simulink model "Vehicle_Model_WIP_V2"  (R2019b)
settings: Solver=FixedStepDiscrete  StartTime=0.0  StopTime=Simulink.t_end  FixedStep=Simulink.dt  RelTol=1e-3
undefined symbols (not defined in the file): BRK, BTRRAD, CHLR, CHRG, DCDC, DiscIntNeverNeededParam, FAN, INV, MTR, PTRAD, PUMP, Settings, TRSM, Vehicle, VHCL, WHL
libraries: simulink x9, EV_cooling x6, EV_VLD x5, EV_ePWT x5
(part 5 of 5)

== system Vehicle_Model_WIP_V2/old cooling/Fan and air for Radiators/Air Flow and Fan Model/Fan Inertia ==
  Max Volumetric flow rate [lpm : Inport
  Discrete-Time Integrator : DiscreteIntegrator  SampleTime=-1  ICPrevOutput=DiscIntNeverNeededParam  ICPrevScaledInput=DiscIntNeverNeededParam
  Divide6 : Product  Inputs=*/
  Divide7 : Product  Inputs=*/
  Divide8 : Product  Inputs=/*
  Subtract : Sum  Inputs=+-
  Tau : Constant  Value=3
  one : Constant
  RAD_dVFan_m3ph : Outport
  wires:
  Discrete-Time Integrator/1 -> RAD_dVFan_m3ph/1, Divide7/1
  Divide8/1 -> Divide6/2
  Tau/1 -> Divide7/2, Divide8/2
  Max Volumetric flow rate [lpm/1 -> Divide6/1
  one/1 -> Divide8/1
  Divide6/1 -> Subtract/1
  Subtract/1 -> Discrete-Time Integrator/1
  Divide7/1 -> Subtract/2

== system Vehicle_Model_WIP_V2/old cooling/Fan and air for Radiators/Air Flow and Fan Model/If Action Subsystem ==
  In1 : Inport
  Action Port : ActionPort  ActionPortLabel=if(u1 == 1)
  Out1 : Outport
  wires:
  In1/1 -> Out1/1

== system Vehicle_Model_WIP_V2/old cooling/Fan and air for Radiators/Air Flow and Fan Model/If Action Subsystem1 ==
  In1 : Inport
  Action Port : ActionPort  ActionPortLabel=else
  Out1 : Outport
  wires:
  In1/1 -> Out1/1

== system Vehicle_Model_WIP_V2/old cooling/PowerTrain Cooling system/Low Temperature Radiator/Radiator Thermal model  ==
  RADBCS_TAirOut_degC : Inport
  RAD_TWtrIn_degC : Inport  Port=2
  RAD_dmAir_kgps : Inport  Port=3
  RAD_dmWtr_kgps : Inport  Port=4
  RAD_UA_WpK : Inport  Port=5
  Air Heat Capacity J/kgK : Lookup_n-D  NumberOfTableDimensions=1  BreakpointsForDimension1=[-40 -30 -20 -10 0 5 10 15 20 25 30 35 40 45 50 60 70 80 90 100]  Table=[1002 1004 1005 1006 1006 1007 1008 1009 1010 1011 1011 1012 1013 1014 1016 1017 1019 1020 1021 1022]  ExtrapMethod=Clip  RndMeth=Simplest  InputSameDT=on
  Constant : Constant  Value=-1
  Constant{1..3,7} (4 alike) : Constant
  Constant4 : Constant  Value=-1
  Constant6 : Constant  Value=-1
  Delay : Delay  DelayLength=1  InitialConditionSource=Input port
      settings: InputPortMap=u0,p4
  Delay1 : Delay  InitialConditionSource=Input port
      settings: InputPortMap=u0,p4
  Divide{1,3,8,10,12,15} (6 alike) : Product  Inputs=*/
  Divide{2,4..7,9,11,13..14,16} (10 alike) : Product  Inputs=**
  Exp : Math  SignedPower=off  SaturateOnIntegerOverflow=on
  Exp1 : Math  SignedPower=off  SaturateOnIntegerOverflow=on
  Exp2 : Math  SignedPower=off  SaturateOnIntegerOverflow=on
  Gain : Gain  Gain=0.5
  Heat Capacity  Water-Glycol 80-20%vol J/kgK : Lookup_n-D  NumberOfTableDimensions=1  BreakpointsForDimension1=[-45.56 -17.78 10 37.77 65.55 93.33 121.11 148.88 176.66]  Table="[3841.6 3888.1  3934.6 3981.1 4027.6 4074.0 4120.5 4167.0 4213.6]"  ExtrapMethod=Clip  RndMeth=Simplest  InputSameDT=on
  If Action Subsystem1 : Subsystem  Commented=on  TreatAsAtomicUnit=on
  Subtract{1..7} (7 alike) : Sum  Inputs=+-
  Subtract8 : Sum
  RAD_TAirOut_degC : Outport  VectorParamsAs1DForOutWhenUnconnected=off
  RAD_TWtrOut_degC : Outport  Port=2  VectorParamsAs1DForOutWhenUnconnected=off
  RAD_TWtrBlk_degC : Outport  Port=3  VectorParamsAs1DForOutWhenUnconnected=off
  RAD_PHeatRej_W : Outport  Port=4  VectorParamsAs1DForOutWhenUnconnected=off
  wires:
  [RAD_TWtrBlk_degC] -> RAD_TWtrBlk_degC/1
  [RAD_TAirOut_degC] -> RAD_TAirOut_degC/1
  [RAD_TWtrOut_degC] -> RAD_TWtrOut_degC/1
  Heat Capacity  Water-Glycol 80-20%vol J/kgK/1 -> [RAD_cpWtr]
  [RAD_TWtrBlk_degC] -> Heat Capacity  Water-Glycol 80-20%vol J/kgK/1
  [RAD_TAirBlk_degC] -> Air Heat Capacity J/kgK/1
  Air Heat Capacity J/kgK/1 -> [RAD_cpAir]
  [RAD_PHeatRej_W] -> RAD_PHeatRej_W/1
  RAD_UA_WpK/1 -> [RAD_UA_WpK]
  RAD_dmAir_kgps/1 -> [RAD_dmAir_kgps]
  RAD_dmWtr_kgps/1 -> [RAD_dmWtr_kgps]
  RADBCS_TAirOut_degC/1 -> [RADBCS_TAirOut_degC]
  RAD_TWtrIn_degC/1 -> [RAD_TWtrIn_degC]
  [RAD_PHeatRej_W] -> Divide13/2
  [RAD_dmWtr_kgps] -> Divide6/1
  Divide9/1 -> [RAD_PHeatRej_W]
  Exp/1 -> Subtract2/2
  [RAD_TAirBlk_degC] -> Subtract5/1
  Divide13/1 -> Subtract5/2
  [tauWtr] -> Divide8/2
  Subtract3/1 -> Divide11/1
  [RAD_TAirBlk_degC] -> Subtract1/1
  Exp1/1 -> Divide11/2
  Constant7/1 -> Divide12/1
  [RAD_TAirBlk_degC] -> Subtract3/1
  Constant2/1 -> Subtract2/1
  Subtract1/1 -> Divide7/2
  [RAD_TWtrIn_degC] -> Subtract1/2
  Constant6/1 -> Divide10/1
  Divide5/1 -> [tauWtr]
  [RAD_TAirBlk_degC] -> Subtract4/1
  [RAD_UA_WpK] -> Divide12/2
  Subtract4/1 -> [RAD_TWtrOut_degC]
  [tauWtr] -> Divide10/2
  Divide3/1 -> Divide5/2
  Divide11/1 -> Subtract4/2
  Divide10/1 -> Exp1/1
  Divide2/1 -> Divide5/1
  [RAD_TWtrIn_degC] -> Delay/2
  Subtract2/1 -> Divide9/2
  Constant/1 -> Divide8/1
  Divide6/1 -> Divide7/1
  Divide7/1 -> Divide9/1
  Divide8/1 -> Exp/1
  [RAD_dmWtr_kgps] -> Divide2/1
  [RAD_cpWtr] -> Divide2/2
  Subtract5/1 -> Delay/1
  [RAD_cpWtr] -> Divide6/2
  [RAD_TWtrIn_degC] -> Subtract3/2
  Divide12/1 -> Divide13/1
  Delay/1 -> [RAD_TWtrBlk_degC]
  [RAD_UA_WpK] -> Divide3/2
  Constant3/1 -> Divide3/1
  Constant1/1 -> Divide15/1
  [RAD_UA_WpK] -> Divide15/2
  [RADBCS_TAirOut_degC] -> Subtract6/2
  [RAD_cpAir] -> Divide14/2
  [RAD_dmAir_kgps] -> Divide14/1
  Divide14/1 -> Divide16/1
  Divide1/1 -> Exp2/1
  Divide4/1 -> Subtract7/2
  Divide15/1 -> Divide16/2
  [tauAir] -> Divide1/2
  Subtract7/1 -> [RAD_TAirOut_degC]
  [RAD_TWtrBlk_degC] -> Subtract7/1
  Divide16/1 -> [tauAir]
  Constant4/1 -> Divide1/1
  [RAD_TWtrBlk_degC] -> Subtract6/1
  Exp2/1 -> Divide4/2
  Subtract6/1 -> Divide4/1
  Delay1/1 -> [RAD_TAirBlk_degC]
  [RADBCS_TAirOut_degC] -> Subtract8/1
  [RAD_TAirOut_degC] -> Subtract8/2
  Subtract8/1 -> Gain/1
  [RADBCS_TAirOut_degC] -> Delay1/2
  Gain/1 -> Delay1/1

== system Vehicle_Model_WIP_V2/VLD/old/OLD VLD/Vehicle Longitudinal Dinamic  Model (No Slip)/Wheel speed Front ==
  Vehicle Actual Speed [km/h] : Inport
  VLD_RWhlFr_m : Inport  Port=2
  Constant : Constant  Value=3.6
  Constant1 : Constant  Value=60
  Constant2 : Constant  Value=pi()
  Constant3 : Constant  Value=2
  Constant4 : Constant
  Divide : Product  Inputs=*/
  Divide1 : Product  Inputs=*/
  Divide2 : Product
  Divide3 : Product  Inputs=*/
  Divide4 : Product
  Max : MinMax  Function=max  Inputs=2
  VLD_nWhlFr_rpm : Outport  VectorParamsAs1DForOutWhenUnconnected=off
  VLD_vWhlFr_mps : Outport  Port=2
  wires:
  Divide/1 -> Divide1/1, [VLD_vWhlFr_mps]
  [VLD_vWhlFr_mps] -> VLD_vWhlFr_mps/1
  VLD_RWhlFr_m/1 -> [VLD_RWhlFr_m]
  Vehicle Actual Speed [km/h]/1 -> [Vehicle_Actual_Speed_kph]
  [Vehicle_Actual_Speed_kph] -> Divide/1
  Constant/1 -> Divide/2
  [VLD_RWhlFr_m] -> Divide1/2
  Divide1/1 -> Divide2/1
  Constant1/1 -> Divide2/2
  Divide2/1 -> Divide3/1
  Divide4/1 -> Divide3/2
  Constant3/1 -> Divide4/1
  Constant2/1 -> Divide4/2
  Divide3/1 -> Max/1
  [VLD_nWhlFr_rpm] -> VLD_nWhlFr_rpm/1
  Max/1 -> [VLD_nWhlFr_rpm]
  Constant4/1 -> Max/2

== system Vehicle_Model_WIP_V2/VLD/old/OLD VLD/Vehicle Longitudinal Dinamic  Model (No Slip)/Wheel speed Rear ==
  Vehicle Actual Speed [km/h] : Inport
  VLD_RWhlRr_m : Inport  Port=2
  Constant : Constant  Value=3.6
  Constant1 : Constant  Value=60
  Constant2 : Constant  Value=pi()
  Constant3 : Constant  Value=2
  Constant4 : Constant
  Divide : Product  Inputs=*/
  Divide1 : Product  Inputs=*/
  Divide2 : Product
  Divide3 : Product  Inputs=*/
  Divide4 : Product
  Max : MinMax  Function=max  Inputs=2
  LVD_nWhlRr_rpm : Outport  VectorParamsAs1DForOutWhenUnconnected=off
  VLD_vWhlRr_mps : Outport  Port=2
  wires:
  [VLD_vWhlRr_mps] -> VLD_vWhlRr_mps/1
  Constant4/1 -> Max/2
  [VLD_nWhlRr_rpm] -> LVD_nWhlRr_rpm/1
  Divide3/1 -> Max/1
  Constant2/1 -> Divide4/2
  Constant3/1 -> Divide4/1
  Divide4/1 -> Divide3/2
  Divide2/1 -> Divide3/1
  Constant1/1 -> Divide2/2
  Divide1/1 -> Divide2/1
  [VLD_RWhlRr_m] -> Divide1/2
  Divide/1 -> Divide1/1, [VLD_vWhlRr_mps]
  Constant/1 -> Divide/2
  [Vehicle_Actual_Speed_kph] -> Divide/1
  Vehicle Actual Speed [km/h]/1 -> [Vehicle_Actual_Speed_kph]
  VLD_RWhlRr_m/1 -> [VLD_RWhlRr_m]
  Max/1 -> [VLD_nWhlRr_rpm]

== system Vehicle_Model_WIP_V2/VLD/old/OLD VLD/Vehicle Longitudinal Dinamic Model (Slip)/Slip Model Front ==
  VLD_vWhl_mps : Inport
  VLD_vVhcl_mps : Inport  Port=2
  Abs : Abs
  Constant3 : Constant  Value=1e-3
  Gain : Gain  Gain=3.6
  Gain1 : Gain  Gain=3.6
  If : If  IfExpression=u1 == 1
  If Action Subsystem : Subsystem  TreatAsAtomicUnit=on
  If Action Subsystem1 : Subsystem  TreatAsAtomicUnit=on
  Merge : Merge
  Relational Operator2 : RelationalOperator  Operator=>  OutDataTypeStr=boolean  RndMeth=Simplest
  Saturatio1 : Saturate  UpperLimit=inf  LowerLimit=1e-3
  Saturatio2 : Saturate  UpperLimit=inf  LowerLimit=1e-3
  Saturatio3 : Saturate  UpperLimit=1  LowerLimit=-1
  Scope2 : Scope
  Slip Calculation2 : Subsystem  Commented=on
  Slip Calculation3 : Subsystem
  Zero : Constant  Value=0  OutDataTypeStr=Inherit: Inherit via back propagation
  slip : Outport
  wires:
  [VLD_rSlip] -> slip/1
  [VLD_vVhcl_mps] -> Gain1/1
  If/2 -> If Action Subsystem1/Action
  Saturatio1/1 -> Slip Calculation3/1(w)
  Saturatio2/1 -> Slip Calculation3/2(v)
  If Action Subsystem/1(Out1) -> Merge/1
  Merge/1 -> Saturatio3/1
  Constant3/1 -> Relational Operator2/2
  Relational Operator2/1 -> If/1
  If Action Subsystem1/1(Out1) -> Merge/2
  Abs/1 -> Relational Operator2/1
  Zero/1 -> If Action Subsystem1/1(In1)  "slip"
  [VLD_vWhl_mps] -> Abs/1, Gain/1
  If/1 -> If Action Subsystem/Action
  Slip Calculation3/1(slip) -> If Action Subsystem/1(In1)
  VLD_vVhcl_mps/1 -> [VLD_vVhcl_mps]
  VLD_vWhl_mps/1 -> [VLD_vWhl_mps]
  Saturatio3/1 -> [VLD_rSlip], Scope2/1
  Gain/1 -> Saturatio1/1
  Gain1/1 -> Saturatio2/1

== system Vehicle_Model_WIP_V2/VLD/old/OLD VLD/Vehicle Longitudinal Dinamic Model (Slip)/Slip Model Rear ==
  VLD_vWhl_mps : Inport
  VLD_vVhcl_mps : Inport  Port=2
  Abs : Abs
  Constant3 : Constant  Value=1e-3
  Gain1 : Gain  Gain=3.6
  Gain2 : Gain  Gain=3.6
  If : If  IfExpression=u1 == 1
  If Action Subsystem : Subsystem  TreatAsAtomicUnit=on
  If Action Subsystem1 : Subsystem  TreatAsAtomicUnit=on
  Merge : Merge
  Relational Operator2 : RelationalOperator  Operator=>  OutDataTypeStr=boolean  RndMeth=Simplest
  Saturatio1 : Saturate  UpperLimit=inf  LowerLimit=1e-3
  Saturatio2 : Saturate  UpperLimit=inf  LowerLimit=1e-3
  Scope2 : Scope
  Scope3 : Scope
  Scope6 : Scope
  Slip Calculation2 : Subsystem  Commented=on
  Slip Calculation3 : Subsystem
  Zero : Constant  Value=0  OutDataTypeStr=Inherit: Inherit via back propagation
  slip : Outport
  wires:
  VLD_vWhl_mps/1 -> [VLD_vWhl_mps]
  VLD_vVhcl_mps/1 -> [VLD_vVhcl_mps]
  Slip Calculation3/1(slip) -> If Action Subsystem/1(In1), Scope3/1
  If/1 -> If Action Subsystem/Action
  [VLD_vWhl_mps] -> Abs/1, Gain1/1
  Zero/1 -> If Action Subsystem1/1(In1)  "slip"
  Abs/1 -> Relational Operator2/1
  If Action Subsystem1/1(Out1) -> Merge/2
  Relational Operator2/1 -> If/1, Scope6/1
  Constant3/1 -> Relational Operator2/2
  If Action Subsystem/1(Out1) -> Merge/1
  Saturatio2/1 -> Slip Calculation3/2(v)
  Saturatio1/1 -> Slip Calculation3/1(w)
  If/2 -> If Action Subsystem1/Action
  [VLD_vVhcl_mps] -> Gain2/1
  [VLD_rSlip] -> slip/1
  Merge/1 -> [VLD_rSlip], Scope2/1
  Gain1/1 -> Saturatio1/1
  Gain2/1 -> Saturatio2/1

== system Vehicle_Model_WIP_V2/VLD/old/OLD VLD/Vehicle Longitudinal Dinamic Model (Slip)/Subsystem2 ==
  rad/s : Inport
  Constant1 : Constant  Value=60
  Constant2 : Constant  Value=pi()
  Constant3 : Constant  Value=2
  Divide2 : Product
  Divide3 : Product  Inputs=*/
  Divide4 : Product
  rpm : Outport
  wires:
  rad/s/1 -> Divide2/1
  Constant2/1 -> Divide4/2
  Divide2/1 -> Divide3/1
  Divide3/1 -> rpm/1
  Constant1/1 -> Divide2/2
  Divide4/1 -> Divide3/2
  Constant3/1 -> Divide4/1

== system Vehicle_Model_WIP_V2/VLD/old/OLD VLD/Vehicle Longitudinal Dinamic Model (Slip)/Subsystem3 ==
  rad/s : Inport
  Constant1 : Constant  Value=60
  Constant2 : Constant  Value=pi()
  Constant3 : Constant  Value=2
  Divide2 : Product
  Divide3 : Product  Inputs=*/
  Divide4 : Product
  rpm : Outport
  wires:
  Constant3/1 -> Divide4/1
  Divide4/1 -> Divide3/2
  Constant1/1 -> Divide2/2
  Divide3/1 -> rpm/1
  Divide2/1 -> Divide3/1
  Constant2/1 -> Divide4/2
  rad/s/1 -> Divide2/1

== system Vehicle_Model_WIP_V2/VLD/old/OLD VLD/Vehicle Longitudinal Dinamic Model (Slip)/Tire Model ==
  VLD_rSlip : Inport
  VLD_WDistr : Inport  Port=2
  1-D Lookup Table : Lookup_n-D  Commented=on  NumberOfTableDimensions=1  BreakpointsForDimension1=-1:0.05:1  Table="[-0.7 -0.71,-0.72,-0.73,-0.75,-0.77,-0.79,-0.81,-0.83,-0.855,-0.88,-0.90,-0.92,-0.94,-0.96,-0.98,-1,-0.97,-0.8,-0.4 0  0.4 0.8 0.97 1 0.98 0.96 0.94 0.92 0.9 0.88 0.855 0.83 0.81 0.79 0.77 0.75 0.73 0.72 0.71 0.7]"  ExtrapMethod=Clip  InternalRulePriority=Speed  RndMeth=Simplest  InputSameDT=on
  1-D Lookup Table1 : Lookup_n-D  BreakpointsForDimension1=WHL.Front.Fz_bp  BreakpointsForDimension2=WHL.Front.slip_bp(13:25)  Table=WHL.Front.mu(:,13:25)  ExtrapMethod=Clip  InternalRulePriority=Speed  RndMeth=Simplest  InputSameDT=on
  Constant3 : Constant  Commented=on  Value=VHCL.Front.Frict_Coeff
  Demux1 : Demux  Commented=on  Outputs=2
  Divide11 : Product  Commented=on
  Gain : Gain  Gain=0.5
  MATLAB Function : MATLAB Function  Commented=on  TreatAsAtomicUnit=on
  MATLAB Function1 : MATLAB Function  Commented=on  TreatAsAtomicUnit=on
  Mux : Mux  Commented=on  Inputs=2
  VLD_mu : Outport
  wires:
  1-D Lookup Table1/1 -> VLD_mu/1
  Demux1/2 -> MATLAB Function1/1(slip)
  Demux1/1 -> MATLAB Function/1(slip)
  Constant3/1 -> Divide11/1
  1-D Lookup Table/1 -> Divide11/2
  MATLAB Function1/1(mu_x) -> Mux/2
  VLD_rSlip/1 -> 1-D Lookup Table1/2
  MATLAB Function/1(mu_x) -> Mux/1
  VLD_WDistr/1 -> Gain/1
  Gain/1 -> 1-D Lookup Table1/1

== system Vehicle_Model_WIP_V2/old cooling/Battery Cooling system/Low Temperature Radiator/Radiator Thermal model /If Action Subsystem ==
  In1 : Inport
  In2 : Inport  Port=2
  In4 : Inport  Port=3
  Action Port : ActionPort  ActionPortLabel=if(u1 ~= 0)
  Out1 : Outport
  Out2 : Outport  Port=2
  Out4 : Outport  Port=3
  wires:
  In1/1 -> Out1/1
  In2/1 -> Out2/1
  In4/1 -> Out4/1

== system Vehicle_Model_WIP_V2/old cooling/Battery Cooling system/Low Temperature Radiator/Radiator Thermal model /If Action Subsystem1 ==
  In1 : Inport
  In2 : Inport  Port=2
  In4 : Inport  Port=3
  Action Port : ActionPort  ActionPortLabel=else
  Out1 : Outport
  Out2 : Outport  Port=2
  Out4 : Outport  Port=3
  wires:
  In4/1 -> Out4/1
  In2/1 -> Out2/1
  In1/1 -> Out1/1

== system Vehicle_Model_WIP_V2/old cooling/PowerTrain Cooling system/Low Temperature Radiator/Radiator Thermal model /If Action Subsystem1 ==
  note: q_dot = UA(TWtrOut - TAirIn) = dmWtr*cpWtr(TWtrIn - TWtrOut)
      | --> TWtrOut = (TWtrIn + (UA/(dmWtr*cpWtr))TAirIn)/(1+UA/(dmWtr*cpWtr))
  RAD_TWtrIn_degC : Inport
  RADBCS_TAirOut_degC : Inport  Port=2
  RAD_UA_WpK : Inport  Port=3
  RAD_dmWtr_kgps : Inport  Port=4
  RAD_cpWtr : Inport  Port=5
  Action Port : ActionPort  ActionPortLabel=else
  Add1 : Sum
  Add3 : Sum  Inputs=-+
  Add4 : Sum
  Add6 : Sum  Inputs=+++
  Constant1 : Constant  Value=273.15
  Constant13 : Constant  Value=273.15
  Constant2 : Constant  Value=273.15
  Constant3 : Constant
  Produt3 : Product  Inputs=**  RndMeth=Zero
  Produt5 : Product  Inputs=*/  RndMeth=Zero
  Produt6 : Product  Inputs=**  RndMeth=Zero
  Produt7 : Product  Inputs=*/  RndMeth=Zero
  RAD_TWtrOut_degC : Outport
  wires:
  RAD_cpWtr/1 -> Produt3/2
  Produt3/1 -> Produt5/2
  Constant2/1 -> Add6/2
  Constant13/1 -> Add3/1
  RAD_dmWtr_kgps/1 -> Produt3/1
  RADBCS_TAirOut_degC/1 -> Add1/1
  Constant1/1 -> Add1/2
  Add4/1 -> Produt7/2  "1+UA/mcw"
  Produt7/1 -> Add3/2
  Add6/1 -> Produt7/1
  Add1/1 -> Produt6/1
  Produt5/1 -> Produt6/2, Add4/1
  Produt6/1 -> Add6/3
  Constant3/1 -> Add4/2
  RAD_TWtrIn_degC/1 -> Add6/1
  Add3/1 -> RAD_TWtrOut_degC/1  "TWtrOut"
  RAD_UA_WpK/1 -> Produt5/1

== system Vehicle_Model_WIP_V2/VLD/old/OLD VLD/Vehicle Longitudinal Dinamic Model (Slip)/Slip Model Front/If Action Subsystem ==
  In1 : Inport
  Action Port : ActionPort  ActionPortLabel=if(u1 == 1)
  Out1 : Outport
  wires:
  In1/1 -> Out1/1

== system Vehicle_Model_WIP_V2/VLD/old/OLD VLD/Vehicle Longitudinal Dinamic Model (Slip)/Slip Model Front/If Action Subsystem1 ==
  In1 : Inport
  Action Port : ActionPort  ActionPortLabel=else
  Out1 : Outport
  wires:
  In1/1 -> Out1/1

== system Vehicle_Model_WIP_V2/VLD/old/OLD VLD/Vehicle Longitudinal Dinamic Model (Slip)/Slip Model Front/Slip Calculation2 ==
  w : Inport
  v : Inport  Port=2
  M : Inport  Port=3
  Abs : Abs
  Constant : Constant  Value=0.01
  Constant1 : Constant  Value=8
  Constant2 : Constant  Value=0
  Constant3 : Constant  Value=15
  Fcn : Fcn  Expr=u(1)/u(2) + (u(2) == 0)*eps- 1
  If : If  IfExpression=u1 == 1
  If Action Subsystem : Subsystem  TreatAsAtomicUnit=on
  If Action Subsystem1 : Subsystem  TreatAsAtomicUnit=on
  Logical Operator : Logic  AllPortsSameDT=off  OutDataTypeStr=boolean
  Merge : Merge
  Mux1 : Mux
  Mux5 : Mux  Inputs=2
  Relational Operator : RelationalOperator  Operator=~=  OutDataTypeStr=boolean  RndMeth=Simplest
  Relational Operator1 : RelationalOperator  Operator=<=  OutDataTypeStr=boolean  RndMeth=Simplest
  Relational Operator2 : RelationalOperator  Operator=>  OutDataTypeStr=boolean  RndMeth=Simplest
  Saturatio1 : Saturate  UpperLimit=inf  LowerLimit=0
  Saturatio2 : Saturate  UpperLimit=1  LowerLimit=-1
  Saturatio3 : Saturate  UpperLimit=1  LowerLimit=-1
  Saturatio5 : Saturate  UpperLimit=inf  LowerLimit=0
  Scope : Scope  NumInputPorts=4
  Scope{1..6} (6 alike) : Scope
  Slip Calculation1 : Subsystem
  Slip Calculation2 : Subsystem
  Slip Calculation3 : Subsystem
  Slip Calculation5 : Subsystem
  Slip Calculation6 : Subsystem
  Subsystem1 : Subsystem
  Subsystem3 : Subsystem
  Switch : Switch  Criteria=u2 > Threshold
  slip : Outport
  wires:
  Mux1/1 -> Scope5/1
  Slip Calculation2/1(slip) -> Mux1/1  "slip"
  Slip Calculation1/1(slip) -> Switch/3, Mux1/2
  v/1 -> Slip Calculation6/2(v), Slip Calculation3/2(v), Slip Calculation5/2(v), Slip Calculation2/2(v), Slip Calculation1/2(v), Saturatio1/1
  Fcn/1 -> Saturatio2/1
  Mux5/1 -> Scope1/1, Fcn/1
  Saturatio5/1 -> Mux5/1
  Saturatio1/1 -> Mux5/2
  Saturatio2/1 -> Mux1/3
  M/1 -> Scope/3, Relational Operator/1
  Relational Operator/1 -> Logical Operator/1
  Relational Operator1/1 -> Logical Operator/2
  Logical Operator/1 -> Scope/1, Switch/2
  Switch/1 -> Scope/2
  Constant/1 -> Switch/1
  Constant1/1 -> Relational Operator1/2
  Constant2/1 -> Relational Operator/2
  If/1 -> If Action Subsystem/Action
  If/2 -> If Action Subsystem1/Action
  Slip Calculation3/1(slip) -> Scope3/1, If Action Subsystem/1(In1)
  If Action Subsystem/1(Out1) -> Merge/1
  If Action Subsystem1/1(Out1) -> Merge/2
  Merge/1 -> Saturatio3/1
  Saturatio3/1 -> slip/1, Scope2/1
  Relational Operator2/1 -> Scope6/1, If/1
  Constant3/1 -> Relational Operator2/2
  Slip Calculation6/1(slip) -> Scope4/1, If Action Subsystem1/1(In1)  "slip"
  Abs/1 -> Relational Operator2/1
  Slip Calculation5/1(slip) -> Mux1/4  "slip"
  w/1 -> Slip Calculation6/1(w), Slip Calculation3/1(w), Scope/4, Relational Operator1/1, Slip Calculation5/1(w), Saturatio5/1, Slip Calculation1/1(w), Slip Calculation2/1(w), Abs/1

== system Vehicle_Model_WIP_V2/VLD/old/OLD VLD/Vehicle Longitudinal Dinamic Model (Slip)/Slip Model Front/Slip Calculation3 ==
  w : Inport
  v : Inport  Port=2
  Product1 : Product  Inputs=/*  SaturateOnIntegerOverflow=on  OutDataTypeStr=Inherit: Same as first input
  Rate Limiter : RateLimiter  RisingSlewLimit=10  FallingSlewLimit=-10  SampleTimeMode=inherited
  Saturatio2 : Saturate  UpperLimit=1  LowerLimit=-1
  Sum : Sum  Inputs=|+-
  slip : Outport
  wires:
  Rate Limiter/1 -> slip/1
  Saturatio2/1 -> Rate Limiter/1
  Product1/1 -> Saturatio2/1
  w/1 -> Product1/1, Sum/1
  v/1 -> Sum/2
  Sum/1 -> Product1/2

== system Vehicle_Model_WIP_V2/VLD/old/OLD VLD/Vehicle Longitudinal Dinamic Model (Slip)/Slip Model Rear/If Action Subsystem ==
  In1 : Inport
  Action Port : ActionPort  ActionPortLabel=if(u1 == 1)
  Out1 : Outport
  wires:
  In1/1 -> Out1/1

== system Vehicle_Model_WIP_V2/VLD/old/OLD VLD/Vehicle Longitudinal Dinamic Model (Slip)/Slip Model Rear/If Action Subsystem1 ==
  In1 : Inport
  Action Port : ActionPort  ActionPortLabel=else
  Out1 : Outport
  wires:
  In1/1 -> Out1/1

== system Vehicle_Model_WIP_V2/VLD/old/OLD VLD/Vehicle Longitudinal Dinamic Model (Slip)/Slip Model Rear/Slip Calculation2 ==
  w : Inport
  v : Inport  Port=2
  M : Inport  Port=3
  Abs : Abs
  Constant : Constant  Value=0.01
  Constant1 : Constant  Value=8
  Constant2 : Constant  Value=0
  Constant3 : Constant  Value=15
  Fcn : Fcn  Expr=u(1)/u(2) + (u(2) == 0)*eps- 1
  If : If  IfExpression=u1 == 1
  If Action Subsystem : Subsystem  TreatAsAtomicUnit=on
  If Action Subsystem1 : Subsystem  TreatAsAtomicUnit=on
  Logical Operator : Logic  AllPortsSameDT=off  OutDataTypeStr=boolean
  Merge : Merge
  Mux1 : Mux
  Mux5 : Mux  Inputs=2
  Relational Operator : RelationalOperator  Operator=~=  OutDataTypeStr=boolean  RndMeth=Simplest
  Relational Operator1 : RelationalOperator  Operator=<=  OutDataTypeStr=boolean  RndMeth=Simplest
  Relational Operator2 : RelationalOperator  Operator=>  OutDataTypeStr=boolean  RndMeth=Simplest
  Saturatio1 : Saturate  UpperLimit=inf  LowerLimit=0
  Saturatio2 : Saturate  UpperLimit=1  LowerLimit=-1
  Saturatio3 : Saturate  UpperLimit=1  LowerLimit=-1
  Saturatio5 : Saturate  UpperLimit=inf  LowerLimit=0
  Scope : Scope  NumInputPorts=4
  Scope{1..6} (6 alike) : Scope
  Slip Calculation1 : Subsystem
  Slip Calculation2 : Subsystem
  Slip Calculation3 : Subsystem
  Slip Calculation5 : Subsystem
  Slip Calculation6 : Subsystem
  Subsystem1 : Subsystem
  Subsystem3 : Subsystem
  Switch : Switch  Criteria=u2 > Threshold
  slip : Outport
  wires:
  w/1 -> Abs/1, Slip Calculation2/1(w), Slip Calculation1/1(w), Saturatio5/1, Slip Calculation5/1(w), Relational Operator1/1, Scope/4, Slip Calculation3/1(w), Slip Calculation6/1(w)
  Slip Calculation5/1(slip) -> Mux1/4  "slip"
  Abs/1 -> Relational Operator2/1
  Slip Calculation6/1(slip) -> If Action Subsystem1/1(In1), Scope4/1  "slip"
  Constant3/1 -> Relational Operator2/2
  Relational Operator2/1 -> If/1, Scope6/1
  Saturatio3/1 -> Scope2/1, slip/1
  Merge/1 -> Saturatio3/1
  If Action Subsystem1/1(Out1) -> Merge/2
  If Action Subsystem/1(Out1) -> Merge/1
  Slip Calculation3/1(slip) -> If Action Subsystem/1(In1), Scope3/1
  If/2 -> If Action Subsystem1/Action
  If/1 -> If Action Subsystem/Action
  Constant2/1 -> Relational Operator/2
  Constant1/1 -> Relational Operator1/2
  Constant/1 -> Switch/1
  Switch/1 -> Scope/2
  Logical Operator/1 -> Switch/2, Scope/1
  Relational Operator1/1 -> Logical Operator/2
  Relational Operator/1 -> Logical Operator/1
  M/1 -> Relational Operator/1, Scope/3
  Saturatio2/1 -> Mux1/3
  Saturatio1/1 -> Mux5/2
  Saturatio5/1 -> Mux5/1
  Mux5/1 -> Fcn/1, Scope1/1
  Fcn/1 -> Saturatio2/1
  v/1 -> Saturatio1/1, Slip Calculation1/2(v), Slip Calculation2/2(v), Slip Calculation5/2(v), Slip Calculation3/2(v), Slip Calculation6/2(v)
  Slip Calculation1/1(slip) -> Mux1/2, Switch/3
  Slip Calculation2/1(slip) -> Mux1/1  "slip"
  Mux1/1 -> Scope5/1

== system Vehicle_Model_WIP_V2/VLD/old/OLD VLD/Vehicle Longitudinal Dinamic Model (Slip)/Slip Model Rear/Slip Calculation3 ==
  w : Inport
  v : Inport  Port=2
  Product1 : Product  Inputs=/*  SaturateOnIntegerOverflow=on  OutDataTypeStr=Inherit: Same as first input
  Rate Limiter : RateLimiter  RisingSlewLimit=10  FallingSlewLimit=-10  SampleTimeMode=inherited
  Saturatio2 : Saturate  UpperLimit=1  LowerLimit=-1
  Sum : Sum  Inputs=|+-
  slip : Outport
  wires:
  v/1 -> Sum/2
  w/1 -> Product1/1, Sum/1
  Product1/1 -> Saturatio2/1
  Saturatio2/1 -> Rate Limiter/1
  Rate Limiter/1 -> slip/1
  Sum/1 -> Product1/2

== system Vehicle_Model_WIP_V2/VLD/old/OLD VLD/Vehicle Longitudinal Dinamic Model (Slip)/Slip Model Front/Slip Calculation2/If Action Subsystem ==
  In1 : Inport
  Action Port : ActionPort
  Out1 : Outport
  wires:
  In1/1 -> Out1/1

== system Vehicle_Model_WIP_V2/VLD/old/OLD VLD/Vehicle Longitudinal Dinamic Model (Slip)/Slip Model Front/Slip Calculation2/If Action Subsystem1 ==
  In1 : Inport
  Action Port : ActionPort
  Out1 : Outport
  wires:
  In1/1 -> Out1/1

== system Vehicle_Model_WIP_V2/VLD/old/OLD VLD/Vehicle Longitudinal Dinamic Model (Slip)/Slip Model Front/Slip Calculation2/Slip Calculation1 ==
  w : Inport
  v : Inport  Port=2
  1-D Lookup Table : Lookup_n-D  NumberOfTableDimensions=1  BreakpointsForDimension1=[0 0.02 0.04 0.06 0.08 0.1]  Table=[2.0 0.09 0.09 0.09 0.09 0.09]  ExtrapMethod=Clip  InternalRulePriority=Speed  RndMeth=Simplest  InputSameDT=on
  Abs : Abs
  Abs2 : Abs
  Add : Sum  Inputs=+-
  Constant : Constant  Value=0.1
  Discrete-Time Integrator : DiscreteIntegrator  SampleTime=-1  ICPrevOutput=DiscIntNeverNeededParam  ICPrevScaledInput=DiscIntNeverNeededParam
  Product1 : Product  Inputs=*/  SaturateOnIntegerOverflow=on  OutDataTypeStr=Inherit: Same as first input
  Product2 : Product  Inputs=**  SaturateOnIntegerOverflow=on  OutDataTypeStr=Inherit: Same as first input
  Product3 : Product  Inputs=*/  SaturateOnIntegerOverflow=on  OutDataTypeStr=Inherit: Same as first input
  Saturatio2 : Saturate  UpperLimit=inf  LowerLimit=1e-6
  Saturatio4 : Saturate  UpperLimit=1  LowerLimit=-1
  Saturatio5 : Saturate  UpperLimit=inf  LowerLimit=1e-6
  Scope : Scope
  Scope1 : Scope
  Subsystem1 : Subsystem
  Subsystem3 : Subsystem
  Sum : Sum  Inputs=|+-
  slip : Outport
  wires:
  Add/1 -> Discrete-Time Integrator/1
  w/1 -> Saturatio5/1
  Product1/1 -> Add/1
  Sum/1 -> Scope1/1, Product1/1
  v/1 -> Saturatio2/1
  Product3/1 -> Product2/1
  Abs/1 -> Product3/1
  Product2/1 -> Add/2
  Discrete-Time Integrator/1 -> Saturatio4/1, Product2/2
  Saturatio5/1 -> Sum/1
  Saturatio2/1 -> Abs/1, Sum/2
  Abs2/1 -> 1-D Lookup Table/1
  Saturatio4/1 -> Scope/1, slip/1, Abs2/1
  Constant/1 -> Product3/2, Product1/2

== system Vehicle_Model_WIP_V2/VLD/old/OLD VLD/Vehicle Longitudinal Dinamic Model (Slip)/Slip Model Front/Slip Calculation2/Slip Calculation2 ==
  w : Inport
  v : Inport  Port=2
  Product1 : Product  Inputs=*/  SaturateOnIntegerOverflow=on  OutDataTypeStr=Inherit: Same as first input
  Rate Limiter : RateLimiter  RisingSlewLimit=10  FallingSlewLimit=-10  SampleTimeMode=inherited
  Saturatio1 : Saturate  UpperLimit=inf  LowerLimit=1e-6
  Saturatio2 : Saturate  UpperLimit=1  LowerLimit=-1
  Saturatio3 : Saturate  UpperLimit=inf  LowerLimit=1e-6
  Sum : Sum  Inputs=|+-
  slip : Outport
  wires:
  Saturatio3/1 -> Sum/2, Product1/2
  Saturatio1/1 -> Sum/1
  w/1 -> Saturatio1/1
  Sum/1 -> Product1/1
  Product1/1 -> Saturatio2/1
  v/1 -> Saturatio3/1
  Saturatio2/1 -> Rate Limiter/1
  Rate Limiter/1 -> slip/1

== system Vehicle_Model_WIP_V2/VLD/old/OLD VLD/Vehicle Longitudinal Dinamic Model (Slip)/Slip Model Front/Slip Calculation2/Slip Calculation3 ==
  w : Inport
  v : Inport  Port=2
  Product1 : Product  Inputs=*/  SaturateOnIntegerOverflow=on  OutDataTypeStr=Inherit: Same as first input
  Rate Limiter : RateLimiter  RisingSlewLimit=10  FallingSlewLimit=-10  SampleTimeMode=inherited
  Saturatio1 : Saturate  UpperLimit=inf  LowerLimit=1e-6
  Saturatio2 : Saturate  UpperLimit=1  LowerLimit=-1
  Saturatio3 : Saturate  UpperLimit=inf  LowerLimit=1e-6
  Sum : Sum  Inputs=|+-
  slip : Outport
  wires:
  Rate Limiter/1 -> slip/1
  Saturatio2/1 -> Rate Limiter/1
  v/1 -> Saturatio3/1
  Product1/1 -> Saturatio2/1
  Sum/1 -> Product1/1
  w/1 -> Saturatio1/1
  Saturatio1/1 -> Sum/1
  Saturatio3/1 -> Product1/2, Sum/2

== system Vehicle_Model_WIP_V2/VLD/old/OLD VLD/Vehicle Longitudinal Dinamic Model (Slip)/Slip Model Front/Slip Calculation2/Slip Calculation5 ==
  w : Inport
  v : Inport  Port=2
  Max : MinMax  Function=max  Inputs=2
  Product1 : Product  Inputs=*/  SaturateOnIntegerOverflow=on  OutDataTypeStr=Inherit: Same as first input
  Rate Limiter : RateLimiter  RisingSlewLimit=10  FallingSlewLimit=-10  SampleTimeMode=inherited
  Saturatio1 : Saturate  UpperLimit=inf  LowerLimit=1e-6
  Saturatio2 : Saturate  UpperLimit=1  LowerLimit=-1
  Saturatio3 : Saturate  UpperLimit=inf  LowerLimit=1e-6
  Sum : Sum  Inputs=|+-
  slip : Outport
  wires:
  Rate Limiter/1 -> slip/1
  Saturatio2/1 -> Rate Limiter/1
  v/1 -> Saturatio3/1
  Product1/1 -> Saturatio2/1
  w/1 -> Saturatio1/1
  Saturatio1/1 -> Max/2, Sum/1
  Saturatio3/1 -> Sum/2, Max/1
  Sum/1 -> Product1/1
  Max/1 -> Product1/2

== system Vehicle_Model_WIP_V2/VLD/old/OLD VLD/Vehicle Longitudinal Dinamic Model (Slip)/Slip Model Front/Slip Calculation2/Slip Calculation6 ==
  w : Inport
  v : Inport  Port=2
  1-D Lookup Table : Lookup_n-D  NumberOfTableDimensions=1  BreakpointsForDimension1=[0 0.02 0.04 0.06 0.08 0.1]  Table=[2.0 0.09 0.09 0.09 0.09 0.09]  ExtrapMethod=Clip  InternalRulePriority=Speed  RndMeth=Simplest  InputSameDT=on
  Abs : Abs
  Abs2 : Abs
  Add : Sum  Inputs=+-
  Constant : Constant  Value=0.2
  Discrete-Time Integrator : DiscreteIntegrator  SampleTime=-1  ICPrevOutput=DiscIntNeverNeededParam  ICPrevScaledInput=DiscIntNeverNeededParam
  Product1 : Product  Inputs=*/  SaturateOnIntegerOverflow=on  OutDataTypeStr=Inherit: Same as first input
  Product2 : Product  Inputs=**  SaturateOnIntegerOverflow=on  OutDataTypeStr=Inherit: Same as first input
  Product3 : Product  Inputs=*/  SaturateOnIntegerOverflow=on  OutDataTypeStr=Inherit: Same as first input
  Saturatio2 : Saturate  UpperLimit=inf  LowerLimit=1e-6
  Saturatio4 : Saturate  UpperLimit=1  LowerLimit=-1
  Saturatio5 : Saturate  UpperLimit=inf  LowerLimit=1e-6
  Scope : Scope
  Scope1 : Scope
  Subsystem1 : Subsystem
  Subsystem3 : Subsystem
  Sum : Sum  Inputs=|+-
  slip : Outport
  wires:
  Constant/1 -> Product1/2, Product3/2
  Saturatio4/1 -> Abs2/1, slip/1, Scope/1
  Abs2/1 -> 1-D Lookup Table/1
  Saturatio2/1 -> Sum/2, Abs/1
  Saturatio5/1 -> Sum/1
  Discrete-Time Integrator/1 -> Product2/2, Saturatio4/1
  Product2/1 -> Add/2
  Abs/1 -> Product3/1
  Product3/1 -> Product2/1
  v/1 -> Saturatio2/1
  Sum/1 -> Product1/1, Scope1/1
  Product1/1 -> Add/1
  w/1 -> Saturatio5/1
  Add/1 -> Discrete-Time Integrator/1

== system Vehicle_Model_WIP_V2/VLD/old/OLD VLD/Vehicle Longitudinal Dinamic Model (Slip)/Slip Model Front/Slip Calculation2/Subsystem1 ==
  In1 : Inport
  DicrFilter1 : Subsystem
  Out1 : Outport
  wires:
  In1/1 -> DicrFilter1/1(u)
  DicrFilter1/1(Deriv) -> Out1/1

== system Vehicle_Model_WIP_V2/VLD/old/OLD VLD/Vehicle Longitudinal Dinamic Model (Slip)/Slip Model Front/Slip Calculation2/Subsystem3 ==
  In1 : Inport
  Add : Sum  Inputs=+-
  Constant : Constant
  Discrete-Time Integrator : DiscreteIntegrator  SampleTime=-1  ICPrevOutput=DiscIntNeverNeededParam  ICPrevScaledInput=DiscIntNeverNeededParam
  Divide : Product  Inputs=*/
  Out1 : Outport
  wires:
  Discrete-Time Integrator/1 -> Out1/1, Add/2
  In1/1 -> Add/1
  Add/1 -> Divide/1
  Divide/1 -> Discrete-Time Integrator/1
  Constant/1 -> Divide/2

== system Vehicle_Model_WIP_V2/VLD/old/OLD VLD/Vehicle Longitudinal Dinamic Model (Slip)/Slip Model Rear/Slip Calculation2/If Action Subsystem ==
  In1 : Inport
  Action Port : ActionPort
  Out1 : Outport
  wires:
  In1/1 -> Out1/1

== system Vehicle_Model_WIP_V2/VLD/old/OLD VLD/Vehicle Longitudinal Dinamic Model (Slip)/Slip Model Rear/Slip Calculation2/If Action Subsystem1 ==
  In1 : Inport
  Action Port : ActionPort
  Out1 : Outport
  wires:
  In1/1 -> Out1/1

== system Vehicle_Model_WIP_V2/VLD/old/OLD VLD/Vehicle Longitudinal Dinamic Model (Slip)/Slip Model Rear/Slip Calculation2/Slip Calculation1 ==
  w : Inport
  v : Inport  Port=2
  1-D Lookup Table : Lookup_n-D  NumberOfTableDimensions=1  BreakpointsForDimension1=[0 0.02 0.04 0.06 0.08 0.1]  Table=[2.0 0.09 0.09 0.09 0.09 0.09]  ExtrapMethod=Clip  InternalRulePriority=Speed  RndMeth=Simplest  InputSameDT=on
  Abs : Abs
  Abs2 : Abs
  Add : Sum  Inputs=+-
  Constant : Constant  Value=0.1
  Discrete-Time Integrator : DiscreteIntegrator  SampleTime=-1  ICPrevOutput=DiscIntNeverNeededParam  ICPrevScaledInput=DiscIntNeverNeededParam
  Product1 : Product  Inputs=*/  SaturateOnIntegerOverflow=on  OutDataTypeStr=Inherit: Same as first input
  Product2 : Product  Inputs=**  SaturateOnIntegerOverflow=on  OutDataTypeStr=Inherit: Same as first input
  Product3 : Product  Inputs=*/  SaturateOnIntegerOverflow=on  OutDataTypeStr=Inherit: Same as first input
  Saturatio2 : Saturate  UpperLimit=inf  LowerLimit=1e-6
  Saturatio4 : Saturate  UpperLimit=1  LowerLimit=-1
  Saturatio5 : Saturate  UpperLimit=inf  LowerLimit=1e-6
  Scope : Scope
  Scope1 : Scope
  Subsystem1 : Subsystem
  Subsystem3 : Subsystem
  Sum : Sum  Inputs=|+-
  slip : Outport
  wires:
  Constant/1 -> Product1/2, Product3/2
  Saturatio4/1 -> Abs2/1, slip/1, Scope/1
  Abs2/1 -> 1-D Lookup Table/1
  Saturatio2/1 -> Sum/2, Abs/1
  Saturatio5/1 -> Sum/1
  Discrete-Time Integrator/1 -> Product2/2, Saturatio4/1
  Product2/1 -> Add/2
  Abs/1 -> Product3/1
  Product3/1 -> Product2/1
  v/1 -> Saturatio2/1
  Sum/1 -> Product1/1, Scope1/1
  Product1/1 -> Add/1
  w/1 -> Saturatio5/1
  Add/1 -> Discrete-Time Integrator/1

== system Vehicle_Model_WIP_V2/VLD/old/OLD VLD/Vehicle Longitudinal Dinamic Model (Slip)/Slip Model Rear/Slip Calculation2/Slip Calculation2 ==
  w : Inport
  v : Inport  Port=2
  Product1 : Product  Inputs=*/  SaturateOnIntegerOverflow=on  OutDataTypeStr=Inherit: Same as first input
  Rate Limiter : RateLimiter  RisingSlewLimit=10  FallingSlewLimit=-10  SampleTimeMode=inherited
  Saturatio1 : Saturate  UpperLimit=inf  LowerLimit=1e-6
  Saturatio2 : Saturate  UpperLimit=1  LowerLimit=-1
  Saturatio3 : Saturate  UpperLimit=inf  LowerLimit=1e-6
  Sum : Sum  Inputs=|+-
  slip : Outport
  wires:
  Rate Limiter/1 -> slip/1
  Saturatio2/1 -> Rate Limiter/1
  v/1 -> Saturatio3/1
  Product1/1 -> Saturatio2/1
  Sum/1 -> Product1/1
  w/1 -> Saturatio1/1
  Saturatio1/1 -> Sum/1
  Saturatio3/1 -> Product1/2, Sum/2

== system Vehicle_Model_WIP_V2/VLD/old/OLD VLD/Vehicle Longitudinal Dinamic Model (Slip)/Slip Model Rear/Slip Calculation2/Slip Calculation3 ==
  w : Inport
  v : Inport  Port=2
  Product1 : Product  Inputs=*/  SaturateOnIntegerOverflow=on  OutDataTypeStr=Inherit: Same as first input
  Rate Limiter : RateLimiter  RisingSlewLimit=10  FallingSlewLimit=-10  SampleTimeMode=inherited
  Saturatio1 : Saturate  UpperLimit=inf  LowerLimit=1e-6
  Saturatio2 : Saturate  UpperLimit=1  LowerLimit=-1
  Saturatio3 : Saturate  UpperLimit=inf  LowerLimit=1e-6
  Sum : Sum  Inputs=|+-
  slip : Outport
  wires:
  Saturatio3/1 -> Sum/2, Product1/2
  Saturatio1/1 -> Sum/1
  w/1 -> Saturatio1/1
  Sum/1 -> Product1/1
  Product1/1 -> Saturatio2/1
  v/1 -> Saturatio3/1
  Saturatio2/1 -> Rate Limiter/1
  Rate Limiter/1 -> slip/1

== system Vehicle_Model_WIP_V2/VLD/old/OLD VLD/Vehicle Longitudinal Dinamic Model (Slip)/Slip Model Rear/Slip Calculation2/Slip Calculation5 ==
  w : Inport
  v : Inport  Port=2
  Max : MinMax  Function=max  Inputs=2
  Product1 : Product  Inputs=*/  SaturateOnIntegerOverflow=on  OutDataTypeStr=Inherit: Same as first input
  Rate Limiter : RateLimiter  RisingSlewLimit=10  FallingSlewLimit=-10  SampleTimeMode=inherited
  Saturatio1 : Saturate  UpperLimit=inf  LowerLimit=1e-6
  Saturatio2 : Saturate  UpperLimit=1  LowerLimit=-1
  Saturatio3 : Saturate  UpperLimit=inf  LowerLimit=1e-6
  Sum : Sum  Inputs=|+-
  slip : Outport
  wires:
  Max/1 -> Product1/2
  Sum/1 -> Product1/1
  Saturatio3/1 -> Max/1, Sum/2
  Saturatio1/1 -> Sum/1, Max/2
  w/1 -> Saturatio1/1
  Product1/1 -> Saturatio2/1
  v/1 -> Saturatio3/1
  Saturatio2/1 -> Rate Limiter/1
  Rate Limiter/1 -> slip/1

== system Vehicle_Model_WIP_V2/VLD/old/OLD VLD/Vehicle Longitudinal Dinamic Model (Slip)/Slip Model Rear/Slip Calculation2/Slip Calculation6 ==
  w : Inport
  v : Inport  Port=2
  1-D Lookup Table : Lookup_n-D  NumberOfTableDimensions=1  BreakpointsForDimension1=[0 0.02 0.04 0.06 0.08 0.1]  Table=[2.0 0.09 0.09 0.09 0.09 0.09]  ExtrapMethod=Clip  InternalRulePriority=Speed  RndMeth=Simplest  InputSameDT=on
  Abs : Abs
  Abs2 : Abs
  Add : Sum  Inputs=+-
  Constant : Constant  Value=0.2
  Discrete-Time Integrator : DiscreteIntegrator  SampleTime=-1  ICPrevOutput=DiscIntNeverNeededParam  ICPrevScaledInput=DiscIntNeverNeededParam
  Product1 : Product  Inputs=*/  SaturateOnIntegerOverflow=on  OutDataTypeStr=Inherit: Same as first input
  Product2 : Product  Inputs=**  SaturateOnIntegerOverflow=on  OutDataTypeStr=Inherit: Same as first input
  Product3 : Product  Inputs=*/  SaturateOnIntegerOverflow=on  OutDataTypeStr=Inherit: Same as first input
  Saturatio2 : Saturate  UpperLimit=inf  LowerLimit=1e-6
  Saturatio4 : Saturate  UpperLimit=1  LowerLimit=-1
  Saturatio5 : Saturate  UpperLimit=inf  LowerLimit=1e-6
  Scope : Scope
  Scope1 : Scope
  Subsystem1 : Subsystem
  Subsystem3 : Subsystem
  Sum : Sum  Inputs=|+-
  slip : Outport
  wires:
  Add/1 -> Discrete-Time Integrator/1
  w/1 -> Saturatio5/1
  Product1/1 -> Add/1
  Sum/1 -> Scope1/1, Product1/1
  v/1 -> Saturatio2/1
  Product3/1 -> Product2/1
  Abs/1 -> Product3/1
  Product2/1 -> Add/2
  Discrete-Time Integrator/1 -> Saturatio4/1, Product2/2
  Saturatio5/1 -> Sum/1
  Saturatio2/1 -> Abs/1, Sum/2
  Abs2/1 -> 1-D Lookup Table/1
  Saturatio4/1 -> Scope/1, slip/1, Abs2/1
  Constant/1 -> Product3/2, Product1/2

== system Vehicle_Model_WIP_V2/VLD/old/OLD VLD/Vehicle Longitudinal Dinamic Model (Slip)/Slip Model Rear/Slip Calculation2/Subsystem1 ==
  In1 : Inport
  DicrFilter1 : Subsystem
  Out1 : Outport
  wires:
  DicrFilter1/1(Deriv) -> Out1/1
  In1/1 -> DicrFilter1/1(u)

== system Vehicle_Model_WIP_V2/VLD/old/OLD VLD/Vehicle Longitudinal Dinamic Model (Slip)/Slip Model Rear/Slip Calculation2/Subsystem3 ==
  In1 : Inport
  Add : Sum  Inputs=+-
  Constant : Constant
  Discrete-Time Integrator : DiscreteIntegrator  SampleTime=-1  ICPrevOutput=DiscIntNeverNeededParam  ICPrevScaledInput=DiscIntNeverNeededParam
  Divide : Product  Inputs=*/
  Out1 : Outport
  wires:
  Constant/1 -> Divide/2
  Divide/1 -> Discrete-Time Integrator/1
  Add/1 -> Divide/1
  In1/1 -> Add/1
  Discrete-Time Integrator/1 -> Add/2, Out1/1

== system Vehicle_Model_WIP_V2/VLD/old/OLD VLD/Vehicle Longitudinal Dinamic Model (Slip)/Slip Model Front/Slip Calculation2/Slip Calculation1/Subsystem1 ==
  In1 : Inport
  DicrFilter1 : Subsystem
  Out1 : Outport
  wires:
  DicrFilter1/1(Deriv) -> Out1/1
  In1/1 -> DicrFilter1/1(u)

== system Vehicle_Model_WIP_V2/VLD/old/OLD VLD/Vehicle Longitudinal Dinamic Model (Slip)/Slip Model Front/Slip Calculation2/Slip Calculation1/Subsystem3 ==
  In1 : Inport
  Add : Sum  Inputs=+-
  Constant : Constant
  Discrete-Time Integrator : DiscreteIntegrator  SampleTime=-1  ICPrevOutput=DiscIntNeverNeededParam  ICPrevScaledInput=DiscIntNeverNeededParam
  Divide : Product  Inputs=*/
  Out1 : Outport
  wires:
  Constant/1 -> Divide/2
  Divide/1 -> Discrete-Time Integrator/1
  Add/1 -> Divide/1
  In1/1 -> Add/1
  Discrete-Time Integrator/1 -> Add/2, Out1/1

== system Vehicle_Model_WIP_V2/VLD/old/OLD VLD/Vehicle Longitudinal Dinamic Model (Slip)/Slip Model Front/Slip Calculation2/Slip Calculation6/Subsystem1 ==
  In1 : Inport
  DicrFilter1 : Subsystem
  Out1 : Outport
  wires:
  In1/1 -> DicrFilter1/1(u)
  DicrFilter1/1(Deriv) -> Out1/1

== system Vehicle_Model_WIP_V2/VLD/old/OLD VLD/Vehicle Longitudinal Dinamic Model (Slip)/Slip Model Front/Slip Calculation2/Slip Calculation6/Subsystem3 ==
  In1 : Inport
  Add : Sum  Inputs=+-
  Constant : Constant
  Discrete-Time Integrator : DiscreteIntegrator  SampleTime=-1  ICPrevOutput=DiscIntNeverNeededParam  ICPrevScaledInput=DiscIntNeverNeededParam
  Divide : Product  Inputs=*/
  Out1 : Outport
  wires:
  Discrete-Time Integrator/1 -> Out1/1, Add/2
  In1/1 -> Add/1
  Add/1 -> Divide/1
  Divide/1 -> Discrete-Time Integrator/1
  Constant/1 -> Divide/2

== system Vehicle_Model_WIP_V2/VLD/old/OLD VLD/Vehicle Longitudinal Dinamic Model (Slip)/Slip Model Front/Slip Calculation2/Subsystem1/DicrFilter1 ==
  u : Inport
  Add : Sum
  Add4 : Sum  Inputs=+-
  Delay : Delay  DelayLength=1
  Product : Product  RndMeth=Zero
  k_FiltFx : Constant  Value=0.05  OutDataTypeStr=Inherit: Inherit via back propagation  SampleTime=-1
  Deriv : Outport  VectorParamsAs1DForOutWhenUnconnected=off
  wires:
  u/1 -> Add4/1
  k_FiltFx/1 -> Product/1
  Add4/1 -> Product/2
  Product/1 -> Add/1
  Add/1 -> Deriv/1, Delay/1
  Delay/1 -> Add4/2, Add/2

== system Vehicle_Model_WIP_V2/VLD/old/OLD VLD/Vehicle Longitudinal Dinamic Model (Slip)/Slip Model Rear/Slip Calculation2/Slip Calculation1/Subsystem1 ==
  In1 : Inport
  DicrFilter1 : Subsystem
  Out1 : Outport
  wires:
  In1/1 -> DicrFilter1/1(u)
  DicrFilter1/1(Deriv) -> Out1/1

== system Vehicle_Model_WIP_V2/VLD/old/OLD VLD/Vehicle Longitudinal Dinamic Model (Slip)/Slip Model Rear/Slip Calculation2/Slip Calculation1/Subsystem3 ==
  In1 : Inport
  Add : Sum  Inputs=+-
  Constant : Constant
  Discrete-Time Integrator : DiscreteIntegrator  SampleTime=-1  ICPrevOutput=DiscIntNeverNeededParam  ICPrevScaledInput=DiscIntNeverNeededParam
  Divide : Product  Inputs=*/
  Out1 : Outport
  wires:
  Discrete-Time Integrator/1 -> Out1/1, Add/2
  In1/1 -> Add/1
  Add/1 -> Divide/1
  Divide/1 -> Discrete-Time Integrator/1
  Constant/1 -> Divide/2

== system Vehicle_Model_WIP_V2/VLD/old/OLD VLD/Vehicle Longitudinal Dinamic Model (Slip)/Slip Model Rear/Slip Calculation2/Slip Calculation6/Subsystem1 ==
  In1 : Inport
  DicrFilter1 : Subsystem
  Out1 : Outport
  wires:
  DicrFilter1/1(Deriv) -> Out1/1
  In1/1 -> DicrFilter1/1(u)

== system Vehicle_Model_WIP_V2/VLD/old/OLD VLD/Vehicle Longitudinal Dinamic Model (Slip)/Slip Model Rear/Slip Calculation2/Slip Calculation6/Subsystem3 ==
  In1 : Inport
  Add : Sum  Inputs=+-
  Constant : Constant
  Discrete-Time Integrator : DiscreteIntegrator  SampleTime=-1  ICPrevOutput=DiscIntNeverNeededParam  ICPrevScaledInput=DiscIntNeverNeededParam
  Divide : Product  Inputs=*/
  Out1 : Outport
  wires:
  Constant/1 -> Divide/2
  Divide/1 -> Discrete-Time Integrator/1
  Add/1 -> Divide/1
  In1/1 -> Add/1
  Discrete-Time Integrator/1 -> Add/2, Out1/1

== system Vehicle_Model_WIP_V2/VLD/old/OLD VLD/Vehicle Longitudinal Dinamic Model (Slip)/Slip Model Rear/Slip Calculation2/Subsystem1/DicrFilter1 ==
  u : Inport
  Add : Sum
  Add4 : Sum  Inputs=+-
  Delay : Delay  DelayLength=1
  Product : Product  RndMeth=Zero
  k_FiltFx : Constant  Value=0.05  OutDataTypeStr=Inherit: Inherit via back propagation  SampleTime=-1
  Deriv : Outport  VectorParamsAs1DForOutWhenUnconnected=off
  wires:
  Delay/1 -> Add/2, Add4/2
  Add/1 -> Delay/1, Deriv/1
  Product/1 -> Add/1
  Add4/1 -> Product/2
  k_FiltFx/1 -> Product/1
  u/1 -> Add4/1

== system Vehicle_Model_WIP_V2/VLD/old/OLD VLD/Vehicle Longitudinal Dinamic Model (Slip)/Slip Model Front/Slip Calculation2/Slip Calculation1/Subsystem1/DicrFilter1 ==
  u : Inport
  Add : Sum
  Add4 : Sum  Inputs=+-
  Delay : Delay  DelayLength=1
  Product : Product  RndMeth=Zero
  k_FiltFx : Constant  Value=0.05  OutDataTypeStr=Inherit: Inherit via back propagation  SampleTime=-1
  Deriv : Outport  VectorParamsAs1DForOutWhenUnconnected=off
  wires:
  Delay/1 -> Add/2, Add4/2
  Add/1 -> Delay/1, Deriv/1
  Product/1 -> Add/1
  Add4/1 -> Product/2
  k_FiltFx/1 -> Product/1
  u/1 -> Add4/1

== system Vehicle_Model_WIP_V2/VLD/old/OLD VLD/Vehicle Longitudinal Dinamic Model (Slip)/Slip Model Front/Slip Calculation2/Slip Calculation6/Subsystem1/DicrFilter1 ==
  u : Inport
  Add : Sum
  Add4 : Sum  Inputs=+-
  Delay : Delay  DelayLength=1
  Product : Product  RndMeth=Zero
  k_FiltFx : Constant  Value=0.05  OutDataTypeStr=Inherit: Inherit via back propagation  SampleTime=-1
  Deriv : Outport  VectorParamsAs1DForOutWhenUnconnected=off
  wires:
  u/1 -> Add4/1
  k_FiltFx/1 -> Product/1
  Add4/1 -> Product/2
  Product/1 -> Add/1
  Add/1 -> Deriv/1, Delay/1
  Delay/1 -> Add4/2, Add/2

== system Vehicle_Model_WIP_V2/VLD/old/OLD VLD/Vehicle Longitudinal Dinamic Model (Slip)/Slip Model Rear/Slip Calculation2/Slip Calculation1/Subsystem1/DicrFilter1 ==
  u : Inport
  Add : Sum
  Add4 : Sum  Inputs=+-
  Delay : Delay  DelayLength=1
  Product : Product  RndMeth=Zero
  k_FiltFx : Constant  Value=0.05  OutDataTypeStr=Inherit: Inherit via back propagation  SampleTime=-1
  Deriv : Outport  VectorParamsAs1DForOutWhenUnconnected=off
  wires:
  u/1 -> Add4/1
  k_FiltFx/1 -> Product/1
  Add4/1 -> Product/2
  Product/1 -> Add/1
  Add/1 -> Deriv/1, Delay/1
  Delay/1 -> Add4/2, Add/2

== system Vehicle_Model_WIP_V2/VLD/old/OLD VLD/Vehicle Longitudinal Dinamic Model (Slip)/Slip Model Rear/Slip Calculation2/Slip Calculation6/Subsystem1/DicrFilter1 ==
  u : Inport
  Add : Sum
  Add4 : Sum  Inputs=+-
  Delay : Delay  DelayLength=1
  Product : Product  RndMeth=Zero
  k_FiltFx : Constant  Value=0.05  OutDataTypeStr=Inherit: Inherit via back propagation  SampleTime=-1
  Deriv : Outport  VectorParamsAs1DForOutWhenUnconnected=off
  wires:
  Delay/1 -> Add/2, Add4/2
  Add/1 -> Delay/1, Deriv/1
  Product/1 -> Add/1
  Add4/1 -> Product/2
  k_FiltFx/1 -> Product/1
  u/1 -> Add4/1

== matlab function Vehicle_Model_WIP_V2/VLD/old/OLD VLD/Vehicle Longitudinal Dinamic Model (Slip)/Tire Model/MATLAB Function ==
  data: slip input; mu_x output
function mu_x  = fcn(slip)


B = 10;
C = 1.9;
D = 1;
E = 0.97;


mu_x = D*sin(C*atan((B*slip-E*(B*slip-atan(B*slip)))));

== matlab function Vehicle_Model_WIP_V2/VLD/old/OLD VLD/Vehicle Longitudinal Dinamic Model (Slip)/Tire Model/MATLAB Function1 ==
  data: slip input; mu_x output
function mu_x  = fcn(slip)


B = 10;
C = 1.9;
D = 1;
E = 0.97;


mu_x = D*sin(C*atan((B*slip-E*(B*slip-atan(B*slip)))));
